simulink model "fault"  (R2018b)
settings: Solver=FixedStepAuto  StartTime=0.0  StopTime=30  FixedStep=0.00001  RelTol=1e-3
values from neighbouring files (symbols this model uses):
  L = P\X    [lmidesigndelta.m]
settings Model: Creator=hjudisssav  LastModifiedBy=hjudisssav

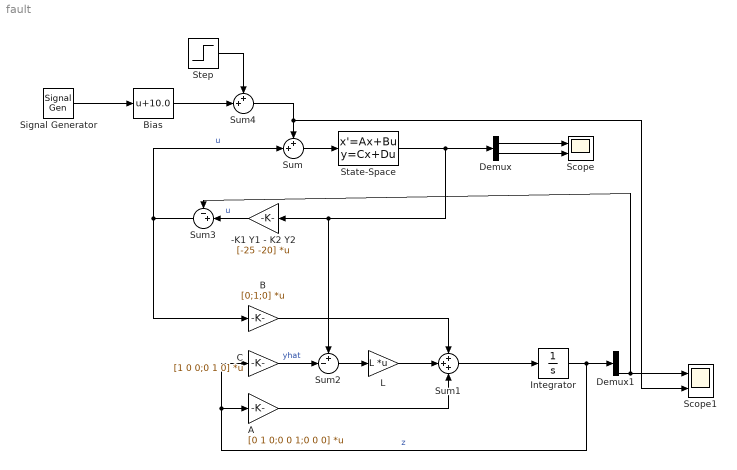
== system fault ==
  -K1 Y1 - K2 Y2 : Gain  Gain=[-25 -20]  Multiplication=Matrix(K*u)
  A : Gain  Gain=[0 1 0;0 0 1;0 0 0]  Multiplication=Matrix(K*u)
  B : Gain  Gain=[0;1;0]  Multiplication=Matrix(K*u)
  Bias : Bias  Bias=10.0
  C : Gain  Gain=[1 0 0;0 1 0]  Multiplication=Matrix(K*u)
  Demux : Demux  Outputs=2
  Demux1 : Demux  Outputs=3
  Integrator : Integrator  InitialCondition=[5;7;0]
  L : Gain  Gain=L  Multiplication=Matrix(K*u)
  Scope : Scope  NumInputPorts=2
  Scope1 : Scope  NumInputPorts=2
  Signal Generator : SignalGenerator  Amplitude=5  Frequency=0.1
  State-Space : StateSpace  A=[0 1;0 0]  B=[0;1]  C=[1 0; 0 1]  D=[0;0]  InitialCondition=[-5;7]
  Step : Step  Time=6  After=10  SampleTime=0
  Sum : Sum  Inputs=++|
  Sum1 : Sum  Inputs=+++
  Sum2 : Sum  Inputs=+-|
  Sum3 : Sum  Inputs=-+|
  Sum4 : Sum  Inputs=++|
  wires:
  State-Space/1 -> Demux/1, Sum2/1, -K1 Y1 - K2 Y2/1
  Sum/1 -> State-Space/1
  Sum3/1 -> Sum/2, B/1  "u"
  Demux/1 -> Scope/1
  Demux/2 -> Scope/2
  Integrator/1 -> Demux1/1, C/1, A/1  "z"
  A/1 -> Sum1/3
  C/1 -> Sum2/2  "yhat"
  B/1 -> Sum1/1
  Sum1/1 -> Integrator/1
  Sum2/1 -> L/1
  L/1 -> Sum1/2
  Demux1/3 -> Sum3/1, Scope1/1
  -K1 Y1 - K2 Y2/1 -> Sum3/2  "u"
  Signal Generator/1 -> Bias/1
  Sum4/1 -> Sum/1, Scope1/2
  Bias/1 -> Sum4/2
  Step/1 -> Sum4/1
